simulink model "nao_linear"  (R2019a)
settings: Solver=VariableStepAuto  StartTime=0.0  StopTime=1500  RelTol=1e-3
settings Model: Creator=josefernandorosaribeiro  LastModifiedBy=josefernandorosaribeiro

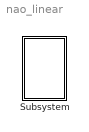
== system nao_linear ==
  Subsystem : Subsystem

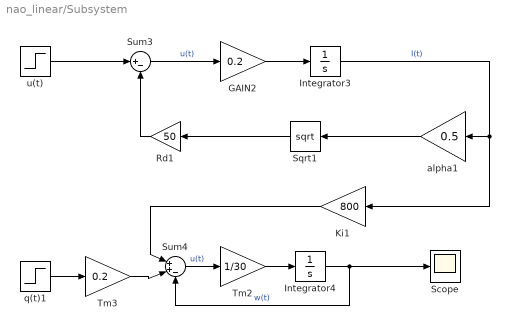
== system nao_linear/Subsystem ==
  GAIN2 : Gain  Gain=0.2
  Integrator3 : Integrator  InitialCondition=0.0072
  Integrator4 : Integrator  InitialCondition=0.0072
  Ki1 : Gain  Gain=800
  Rd1 : Gain  Gain=50
  Scope : Scope
  Sqrt1 : Sqrt  SaturateOnIntegerOverflow=on
  Sum3 : Sum  Inputs=|+-
  Sum4 : Sum  Inputs=|++-
  Tm2 : Gain  Gain=1/30
  Tm3 : Gain  Gain=0.2
  alpha1 : Gain  Gain=0.5
  q(t)1 : Step  Before=5  After=5  SampleTime=0
  u(t) : Step  Before=1  After=5  SampleTime=0
  wires:
  Rd1/1 -> Sum3/2
  GAIN2/1 -> Integrator3/1
  Sum4/1 -> Tm2/1  "u(t)"
  Tm3/1 -> Sum4/2
  Sqrt1/1 -> Rd1/1
  u(t)/1 -> Sum3/1
  Tm2/1 -> Integrator4/1
  Integrator3/1 -> Ki1/1, alpha1/1  "I(t)"
  Ki1/1 -> Sum4/1
  Integrator4/1 -> Sum4/3, Scope/1  "w(t)"
  q(t)1/1 -> Tm3/1
  alpha1/1 -> Sqrt1/1
  Sum3/1 -> GAIN2/1  "u(t)"
